simulink model "beta_hat"  (R2015b)
settings: Solver=VariableStepAuto  StartTime=0.0  StopTime=10.0  RelTol=1e-3
settings Model: Creator=yuji  LastModifiedBy=yuji

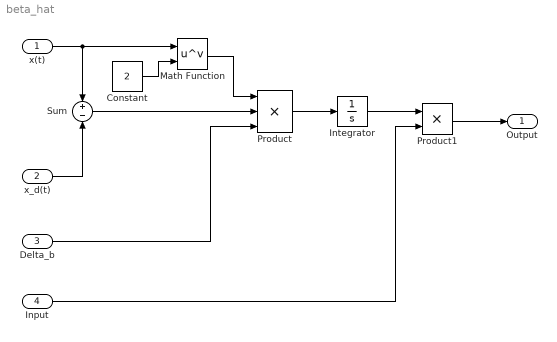
== system beta_hat ==
  x(t) : Inport
  x_d(t) : Inport  Port=2
  Delta_b : Inport  Port=3
  Input : Inport  Port=4
  Constant : Constant  Value=2
  Integrator : Integrator
  Math Function : Math  Operator=pow  SaturateOnIntegerOverflow=on
  Product : Product  Inputs=3
  Product1 : Product
  Sum : Sum  Inputs=+|-
  Output : Outport
  wires:
  x(t)/1 -> Math Function/1, Sum/1
  x_d(t)/1 -> Sum/2
  Sum/1 -> Product/2
  Delta_b/1 -> Product/3
  Product/1 -> Integrator/1
  Integrator/1 -> Product1/1
  Product1/1 -> Output/1
  Input/1 -> Product1/2
  Constant/1 -> Math Function/2
  Math Function/1 -> Product/1
